simulink model "Hunter_gazebo_sub"  (R2023a)
settings: Solver=ode3  StartTime=0.0  StopTime=inf  FixedStep=0.05  RelTol=1e-3  EnableMultiTasking=on
InitFcn:
  | rosshutdown
  | 
  | rosinit("http://localhost:11311")
  | 
  | load('myfcn.mat');
model workspace (MAT data in the model file):
  SL_ROS_VariableLengthArrays_MaxSizes.CommonInfo.ArrayTruncateAction = 'EmitWarning'
  SL_ROS_VariableLengthArrays_MaxSizes.MsgTypeMap = containers.Map
  SL_ROS_VariableLengthArrays_MaxSizes.MsgTypeMap.serialization.keys = {'cob_object_detection_msgs/Detection', 'cob_object_detection_msgs/DetectionArray', 'cob_perception_msgs/DetectionArray', 'gazebo_msgs/ModelStates', 'sensor_msgs/PointCloud2'}
  SL_ROS_VariableLengthArrays_MaxSizes.MsgTypeMap.serialization.values{1}(1).PropertyName = 'Detector'
  SL_ROS_VariableLengthArrays_MaxSizes.MsgTypeMap.serialization.values{1}(1).DataType = 'uint8'
  SL_ROS_VariableLengthArrays_MaxSizes.MsgTypeMap.serialization.values{1}(1).MaxLength = 128
  SL_ROS_VariableLengthArrays_MaxSizes.MsgTypeMap.serialization.values{1}(2).PropertyName = 'Label'
  SL_ROS_VariableLengthArrays_MaxSizes.MsgTypeMap.serialization.values{1}(2).DataType = 'uint8'
  SL_ROS_VariableLengthArrays_MaxSizes.MsgTypeMap.serialization.values{1}(2).MaxLength = 128
  SL_ROS_VariableLengthArrays_MaxSizes.MsgTypeMap.serialization.values{2}.PropertyName = 'Detections'
  SL_ROS_VariableLengthArrays_MaxSizes.MsgTypeMap.serialization.values{2}.DataType = 'cob_object_detection_msgs/Detection'
  SL_ROS_VariableLengthArrays_MaxSizes.MsgTypeMap.serialization.values{2}.MaxLength = 100
  SL_ROS_VariableLengthArrays_MaxSizes.MsgTypeMap.serialization.values{3}.PropertyName = 'Detections'
  SL_ROS_VariableLengthArrays_MaxSizes.MsgTypeMap.serialization.values{3}.DataType = 'cob_perception_msgs/Detection'
  SL_ROS_VariableLengthArrays_MaxSizes.MsgTypeMap.serialization.values{3}.MaxLength = 50
  SL_ROS_VariableLengthArrays_MaxSizes.MsgTypeMap.serialization.values{4}(1).PropertyName = 'Name'
  SL_ROS_VariableLengthArrays_MaxSizes.MsgTypeMap.serialization.values{4}(1).DataType = 'std_msgs/String'
  SL_ROS_VariableLengthArrays_MaxSizes.MsgTypeMap.serialization.values{4}(1).MaxLength = 266
  SL_ROS_VariableLengthArrays_MaxSizes.MsgTypeMap.serialization.values{4}(2).PropertyName = 'Pose'
  SL_ROS_VariableLengthArrays_MaxSizes.MsgTypeMap.serialization.values{4}(2).DataType = 'geometry_msgs/Pose'
  SL_ROS_VariableLengthArrays_MaxSizes.MsgTypeMap.serialization.values{4}(2).MaxLength = 350
  SL_ROS_VariableLengthArrays_MaxSizes.MsgTypeMap.serialization.values{4}(3).PropertyName = 'Twist'
  SL_ROS_VariableLengthArrays_MaxSizes.MsgTypeMap.serialization.values{4}(3).DataType = 'geometry_msgs/Twist'
  SL_ROS_VariableLengthArrays_MaxSizes.MsgTypeMap.serialization.values{4}(3).MaxLength = 350
  SL_ROS_VariableLengthArrays_MaxSizes.MsgTypeMap.serialization.values{5}(1).PropertyName = 'Data'
  SL_ROS_VariableLengthArrays_MaxSizes.MsgTypeMap.serialization.values{5}(1).DataType = 'uint8'
  SL_ROS_VariableLengthArrays_MaxSizes.MsgTypeMap.serialization.values{5}(1).MaxLength = 1050000
  SL_ROS_VariableLengthArrays_MaxSizes.MsgTypeMap.serialization.values{5}(2).PropertyName = 'Fields'
  SL_ROS_VariableLengthArrays_MaxSizes.MsgTypeMap.serialization.values{5}(2).DataType = 'sensor_msgs/PointField'
  SL_ROS_VariableLengthArrays_MaxSizes.MsgTypeMap.serialization.values{5}(2).MaxLength = 1000
  SL_ROS_VariableLengthArrays_MaxSizes.MsgTypeMap.serialization.uniformity = 0
  SL_ROS_VariableLengthArrays_MaxSizes.MsgTypeMap.serialization.keyType = 'char'
  SL_ROS_VariableLengthArrays_MaxSizes.MsgTypeMap.serialization.valueType = 'any'
values from neighbouring files (symbols this model uses):
  roi = [0, 7, -7, 7, -1, 2]    [TrackExample_sim.m]
undefined symbols (not defined in the file or in its folder): Angular, Linear
libraries: robotlib x7, slpidlib x2, slctrlblks x1, robotalgslib x1, mobileRoboticsLib x1, robotcorelib x1
settings Model: Creator=aiv_  LastModifiedBy=aiv
settings SolverCC: AutoInsertRateTranBlk=on
settings DataIOCC: SaveFormat=Array  ReturnWorkspaceOutputs=off
settings OptimizationCC: EnhancedBackFolding=on  PassReuseOutputArgsAs=Individual arguments  StateBitsets=on  DataBitsets=on  ZeroExternalMemoryAtStartup=off  ZeroInternalMemoryAtStartup=off  NoFixptDivByZeroProtection=on  LifeSpan=1  MaxStackSize=64  OptimizeBlockOrder=speed  DifferentSizesBufferReuse=on  EfficientTunableParamExpr=on
settings DebuggingCC: ParameterTunabilityLossMsg=error
settings HardwareCC: ProdBitPerPointer=32  ProdBitPerSizeT=32  ProdBitPerPtrDiffT=32  ProdLargestAtomicFloat=None  ProdWordSize=32  ProdHWDeviceType=Custom Processor->Custom Processor
settings ModelReferenceCC: PropagateSignalLabelsOutOfModel=off
settings SFSimCC: SimTargetLang=C++
settings RTWCC: Description=Embedded Coder  SystemTargetFile=ert.tlc  HardwareBoard=Robot Operating System (ROS)  TLCOptions=-p0 -aRateBasedStepFcn=0  TemplateMakefile=ert_default_tmf  GenerateReport=on  RTWVerbose=off  Toolchain=Catkin  IncludeHyperlinkInReport=on  LaunchReport=on  TargetLang=C++
settings CodeAppCC: ForceParamTrailComments=on  IgnoreCustomStorageClasses=off  OperatorAnnotations=on  SimulinkDataObjDesc=on  SFDataObjDesc=on  CustomSymbolStrGlobalVar=rt$N$M  CustomSymbolStrType=$N$M  CustomSymbolStrFcn=$N$M$F  CustomSymbolStrMacro=$N$M  InsertBlockDesc=on
settings ERTTargetCC: CodeReplacementLibrary=GNU C99 extensions  SuppressErrorStatus=on  CodeInterfacePackaging=C++ class  SupportVariableSizeSignals=on  RootIOFormat=Structure reference  ERTCustomFileTemplate=example_file_process.tlc

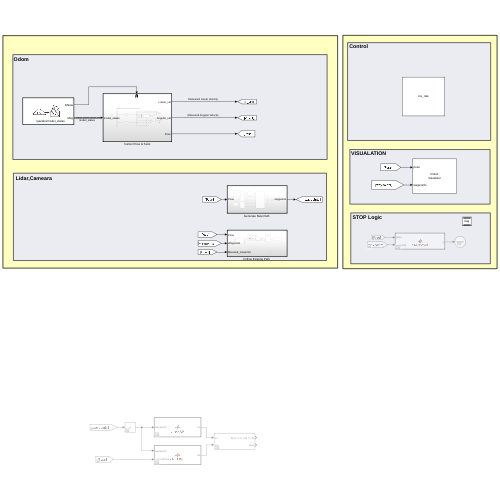
[thumbnail: Simulink's stored preview of the top-level diagram]
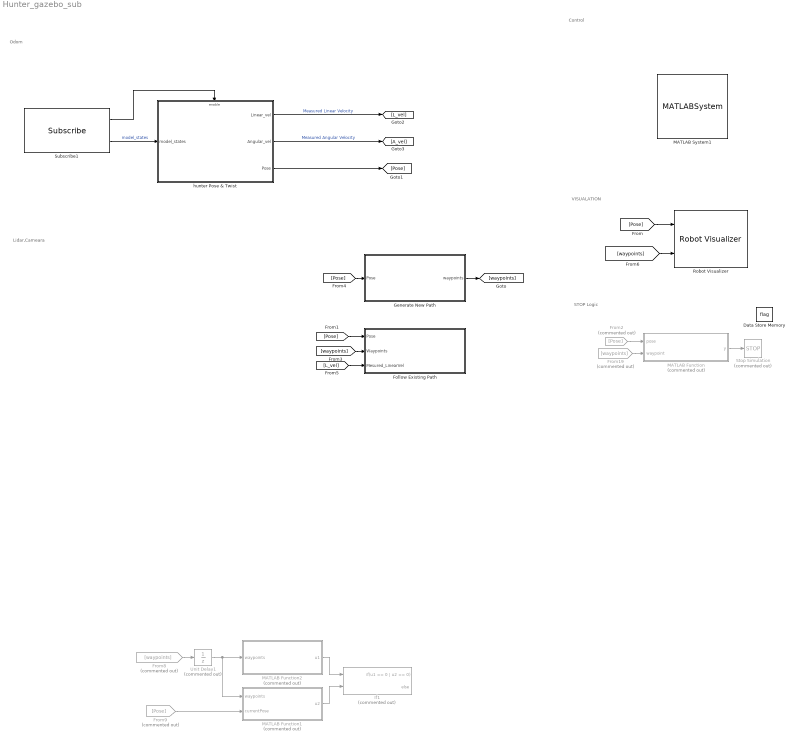
== system Hunter_gazebo_sub ==
  note: VISUALATION
  note: STOP Logic
  note: Odom
  note: Control
  note: Lidar,Cameara
  Data Store Memory : DataStoreMemory  DataStoreName=flag  WriteAfterWriteMsg=warning  ShowAdditionalParam=off  OutDataTypeStr=double
  "Follow Existing Path " : Subsystem  TreatAsAtomicUnit=on
  From19 : From  Commented=on  GotoTag=waypoints
  From2 : From  Commented=on  GotoTag=Pose
  From8 : From  Commented=on  GotoTag=waypoints
  From9 : From  Commented=on  GotoTag=Pose
  "Generate New Path " : Subsystem  TreatAsAtomicUnit=on
  If1 : If  Commented=on  NumInputs=2  IfExpression=u1 == 0 | u2 == 0
  MATLAB Function : MATLAB Function  Commented=on  TreatAsAtomicUnit=on
  MATLAB Function1 : MATLAB Function  Commented=on  TreatAsAtomicUnit=on
  MATLAB Function2 : MATLAB Function  Commented=on  TreatAsAtomicUnit=on
  MATLAB System1 : MATLABSystem  System=ros_rate  RATE=[20]  SimulateUsing=Code generation
      mask Type: ros_rate
      mask Display: disp('ros_rate');
  Robot Visualizer : mobileRoboticsLib/Environments/Robot Visualizer  robotRadius=0  showTrajectory=on  hasWaypoints=on  hasLidar=off  sensorOffset=[ 0, 0 ]  scanAngles=[ -pi/4, 0, pi/4 ]  hasObjDetector=off  objDetectorOffset=[ 0, 0 ]  objDetectorAngle=0  objDetectorFOV=pi/4  objDetectorMaxRange=5  objectColors=[ 1, 0, 0; 0, 1, 0; 0, 0, 1 ]  objectMarkers=s
  Stop Simulation : Stop  Commented=on
  Subscribe1 : robotlib/Subscribe  topicSource=Select from ROS network  topic=/gazebo/model_states  messageType=gazebo_msgs/ModelStates  SampleTime=-1  legacyBusStruct=off  messageQueueLength=1
  Unit Delay1 : UnitDelay  Commented=on  SampleTime=-1  HasFrameUpgradeWarning=on
  hunter Pose & Twist : Subsystem
  wires:
  Subscribe1/1 -> hunter Pose & Twist/Enable
  Subscribe1/2 -> hunter Pose & Twist/1(model_states)  "model_states"
  [waypoints] -> Robot Visualizer/2
  [Pose] -> Robot Visualizer/1
  From2/1 -> MATLAB Function/1(pose)
  MATLAB Function/1(y) -> Stop Simulation/1
  hunter Pose & Twist/1(Linear_vel) -> [L_vel]  "Measured Linear Velocity"
  hunter Pose & Twist/2(Angular_vel) -> [A_vel]  "Measured Angular Velocity"
  From19/1 -> MATLAB Function/2(waypoint)
  [Pose] -> "Generate New Path "/1(Pose)
  "Generate New Path "/1(waypoints) -> [waypoints]
  [Pose] -> "Follow Existing Path "/1(Pose)
  [waypoints] -> "Follow Existing Path "/2(Waypoints)
  [L_vel] -> "Follow Existing Path "/3(Mesured_LinearVel)
  hunter Pose & Twist/3(Pose) -> [Pose]
  MATLAB Function1/1(u2) -> If1/2
  From9/1 -> MATLAB Function1/2(currentPose)
  MATLAB Function2/1(u1) -> If1/1
  Unit Delay1/1 -> MATLAB Function1/1(waypoints), MATLAB Function2/1(waypoints)
  From8/1 -> Unit Delay1/1

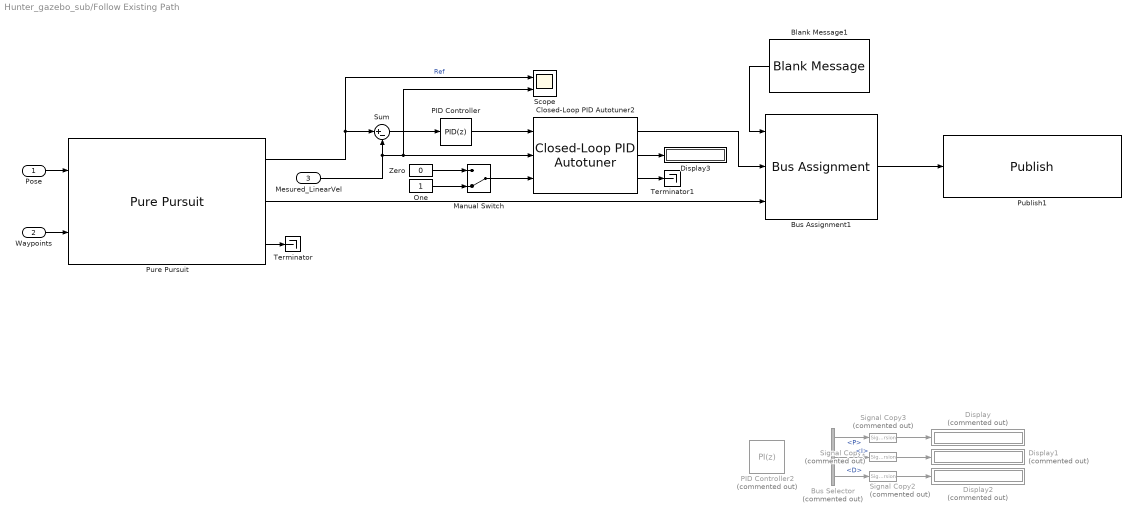
== system Hunter_gazebo_sub/Follow Existing Path  ==
  Pose : Inport
  Waypoints : Inport  Port=2
  Mesured_LinearVel : Inport  Port=3
  Blank Message1 : robotlib/Blank Message  messageClass=Message  entityType=geometry_msgs/Twist  messageType=geometry_msgs/Twist  SampleTime=inf  legacyBusStruct=off
  Bus Assignment1 : BusAssignment  AssignedSignals=Linear.X,Angular.Z
  Bus Selector : BusSelector  Commented=on  OutputSignals=P,I,D
  Closed-Loop PID Autotuner2 : slctrlblks/Closed-Loop PID Autotuner  PIDType=PID  PIDForm=Parallel  TimeDomain=discrete-time  DiscreteTs=0.05  TuningTs=0.2  UseTuningTs=off  IntegratorFormula=Forward Euler  FilterFormula=Forward Euler  ContinuousTs=0.02  Bandwidth=1  UseExternalWC=off  TargetPM=60  UseExternalPM=off  UseExternalAchievedPM=off  ExperimentMode=Superposition  PlantType=Stable  PlantSign=Positive  AmpSine=0.01  UseExternalAmpSine=off  UseExternalFRD=off  UseExternalU0=off  UseCompanion=off  NotDeployTuningModule=off  UsePLCCoder=off  OutputMode=control action + perturbation  BlockDataType=double  UseConnectedPID=on  blockpath=[]  tunedP=0  tunedI=0  tunedD=0  tunedN=100  tunedPM=0  EstimationWindowSize=3  UseExternalTuningParams=off  SingleMultiRateVariant=SingleSamplingRate  NumEstimationPeriods=4  NumSettlingPeriods=2  ExperimentModeVariant=VariantSuperimposed  OutputChoice=VariantCandD
  Display : Display  Commented=on
  Display1 : Display  Commented=on
  Display2 : Display  Commented=on
  Display3 : Display
  Manual Switch : ManualSwitch  CurrentSetting=0
  One : Constant  OutDataTypeStr=Inherit: Inherit via back propagation
  PID Controller : slpidlib/PID Controller  Controller=PID  Form=Parallel  TimeDomain=Discrete-time  UseExternalTs=off  SampleTime=-1  IntegratorMethod=Forward Euler  FilterMethod=Forward Euler  ControllerParametersSource=internal  P=1  I=1  UseKiTs=off  D=0  N=100  UseFilter=on  TunerSelectOption=Transfer Function Based (PID Tuner App)  InitialConditionSource=internal  InitialConditionForIntegrator=0  InitialConditionForFilter=0  DifferentiatorICPrevScaledInput=0  ExternalReset=none  TrackingMode=off  Kt=1  LimitOutput=off  SatLimitsSource=internal  UpperSaturationLimit=inf  LowerSaturationLimit=-inf  LinearizeAsGain=on  AntiWindupMode=none  Kb=1  LimitIntegrator=off  UpperIntegratorSaturationLimit=inf  LowerIntegratorSaturationLimit=-inf  POutMin=[]  POutMax=[]  IOutMin=[]  IOutMax=[]  DOutMin=[]  DOutMax=[]  NOutMin=[]  NOutMax=[]  SumOutMin=[]  SumOutMax=[]  SaturationOutMin=[]  SaturationOutMax=[]  PParamMin=[]  PParamMax=[]  IParamMin=[]  IParamMax=[]  DParamMin=[]  DParamMax=[]  NParamMin=[]  NParamMax=[]  KbParamMin=[]  KbParamMax=[]  KtParamMin=[]  KtParamMax=[]  KbOutMin=[]  KbOutMax=[]  KtOutMin=[]  KtOutMax=[]  IntegratorOutMin=[]  IntegratorOutMax=[]  FilterOutMin=[]  FilterOutMax=[]  SumI1OutMin=[]  SumI1OutMax=[]  SumI2OutMin=[]  SumI2OutMax=[]  SumI3OutMin=[]  SumI3OutMax=[]  SumI4OutMin=[]  SumI4OutMax=[]  SumDOutMin=[]  SumDOutMax=[]  DifferentiatorOutMin=[]  DifferentiatorOutMax=[]  FilterDiffOutCoefMin=[]  FilterDiffOutCoefMax=[]  ReciprocalOutMin=[]  ReciprocalOutMax=[]  SumDenOutMin=[]  SumDenOutMax=[]  SumNumOutMin=[]  SumNumOutMax=[]  DivideOutMin=[]  DivideOutMax=[]  UdiffTsProdOutMin=[]  UdiffTsProdOutMax=[]  NTsProdOutMin=[]  NTsProdOutMax=[]  UintegralTsProdOutMin=[]  UintegralTsProdOutMax=[]  UngainTsProdOutMin=[]  UngainTsProdOutMax=[]  ClampingZeroOutDataTypeStr=Inherit: Inherit via back propagation  ClampingZeroOutMin=[]  ClampingZeroOutMax=[]  FilterDenConstantOutDataTypeStr=Inherit: Inherit via back propagation  FilterDenConstantOutMin=[]  FilterDenConstantOutMax=[]  PCopyOutDataTypeStr=Inherit: Inherit via back propagation  PCopyOutMin=[]  PCopyOutMax=[]  NCopyOutDataTypeStr=Inherit: Inherit via back propagation  NCopyOutMin=[]  NCopyOutMax=[]  IntegratorContinuousStateAttributes=''  IntegratorStateMustResolveToSignalObject=off  IntegratorRTWStateStorageClass=Auto  FilterContinuousStateAttributes=''  FilterStateMustResolveToSignalObject=off  FilterRTWStateStorageClass=Auto  ParallelPVariant=InternalParameters  IdealPVariant=Disabled  IVariant=InternalParameters  DVariant=InternalParameters  IntegratorVariant=Discrete  SatVariant=Disabled  AWVariant=Passthrough  PCopyVariant=Disabled  TRVariant=Disabled  FdbkBlocksVariant=Forward  IdealPFdbkVariant=Disabled  SatFdbkVariant=Disabled  DerivativeFilterVariant=ForwardEulerFilter  NVariant=InternalParameters  NCopyVariant=Disabled  FilterICVariant=InternalICsFilter  IntegratorICVariant=InternalICs  ExternalResetVariant=Disabled  TRSumVariant=Passthrough  SumFdbkVariant=Disabled  SumVariant=Sum_PID  TsampFilterVariant=InternalTs  TsampNgainVariant=Passthrough  TsampIntegralVariant=Disabled_SignalSpec  ExternalSaturationOutDataTypeStr=Inherit: Same as second input
  PID Controller2 : slpidlib/PID Controller  Commented=on  Controller=PI  Form=Parallel  TimeDomain=Discrete-time  UseExternalTs=off  SampleTime=-1  IntegratorMethod=Forward Euler  FilterMethod=Forward Euler  ControllerParametersSource=internal  P=0.6  I=1  UseKiTs=off  D=0.001  N=50  UseFilter=on  TunerSelectOption=Transfer Function Based (PID Tuner App)  InitialConditionSource=internal  InitialConditionForIntegrator=0  InitialConditionForFilter=0  DifferentiatorICPrevScaledInput=0  ExternalReset=none  TrackingMode=off  Kt=1  LimitOutput=off  SatLimitsSource=internal  UpperSaturationLimit=inf  LowerSaturationLimit=-inf  LinearizeAsGain=on  AntiWindupMode=none  Kb=1  LimitIntegrator=off  UpperIntegratorSaturationLimit=inf  LowerIntegratorSaturationLimit=-inf  POutMin=[]  POutMax=[]  IOutMin=[]  IOutMax=[]  DOutMin=[]  DOutMax=[]  NOutMin=[]  NOutMax=[]  SumOutMin=[]  SumOutMax=[]  SaturationOutMin=[]  SaturationOutMax=[]  PParamMin=[]  PParamMax=[]  IParamMin=[]  IParamMax=[]  DParamMin=[]  DParamMax=[]  NParamMin=[]  NParamMax=[]  KbParamMin=[]  KbParamMax=[]  KtParamMin=[]  KtParamMax=[]  KbOutMin=[]  KbOutMax=[]  KtOutMin=[]  KtOutMax=[]  IntegratorOutMin=[]  IntegratorOutMax=[]  FilterOutMin=[]  FilterOutMax=[]  SumI1OutMin=[]  SumI1OutMax=[]  SumI2OutMin=[]  SumI2OutMax=[]  SumI3OutMin=[]  SumI3OutMax=[]  SumI4OutMin=[]  SumI4OutMax=[]  SumDOutMin=[]  SumDOutMax=[]  DifferentiatorOutMin=[]  DifferentiatorOutMax=[]  FilterDiffOutCoefMin=[]  FilterDiffOutCoefMax=[]  ReciprocalOutMin=[]  ReciprocalOutMax=[]  SumDenOutMin=[]  SumDenOutMax=[]  SumNumOutMin=[]  SumNumOutMax=[]  DivideOutMin=[]  DivideOutMax=[]  UdiffTsProdOutMin=[]  UdiffTsProdOutMax=[]  NTsProdOutMin=[]  NTsProdOutMax=[]  UintegralTsProdOutMin=[]  UintegralTsProdOutMax=[]  UngainTsProdOutMin=[]  UngainTsProdOutMax=[]  ClampingZeroOutDataTypeStr=Inherit: Inherit via back propagation  ClampingZeroOutMin=[]  ClampingZeroOutMax=[]  FilterDenConstantOutDataTypeStr=Inherit: Inherit via back propagation  FilterDenConstantOutMin=[]  FilterDenConstantOutMax=[]  PCopyOutDataTypeStr=Inherit: Inherit via back propagation  PCopyOutMin=[]  PCopyOutMax=[]  NCopyOutDataTypeStr=Inherit: Inherit via back propagation  NCopyOutMin=[]  NCopyOutMax=[]  IntegratorContinuousStateAttributes=''  IntegratorStateMustResolveToSignalObject=off  IntegratorRTWStateStorageClass=Auto  FilterContinuousStateAttributes=''  FilterStateMustResolveToSignalObject=off  FilterRTWStateStorageClass=Auto  ParallelPVariant=InternalParameters  IdealPVariant=Disabled  IVariant=InternalParameters  DVariant=Disabled  IntegratorVariant=Discrete  SatVariant=Disabled  AWVariant=Passthrough  PCopyVariant=Disabled  TRVariant=Disabled  FdbkBlocksVariant=Forward  IdealPFdbkVariant=Disabled  SatFdbkVariant=Disabled  DerivativeFilterVariant=Disabled  NVariant=Disabled  NCopyVariant=Disabled_SignalSpec  FilterICVariant=Disabled  IntegratorICVariant=InternalICs  ExternalResetVariant=Disabled  TRSumVariant=Passthrough  SumFdbkVariant=Disabled  SumVariant=Sum_PI  TsampFilterVariant=InternalTs  TsampNgainVariant=Passthrough  TsampIntegralVariant=Disabled_SignalSpec  ExternalSaturationOutDataTypeStr=Inherit: Same as second input
  Publish1 : robotlib/Publish  topicSource=Select from ROS network  topic=/ackermann_steering_controller/cmd_vel  messageType=geometry_msgs/Twist  legacyBusStruct=off  messageQueueLength=1
  Pure Pursuit : robotalgslib/Pure Pursuit  DesiredLinearVelocity=1.5  MaxAngularVelocity=2  LookaheadDistance=1.3  TargetDirPort=on  SimulateUsing=Code generation
      settings: LibrarySourceBlock=navlib/Control Algorithms/Pure Pursuit
  Scope : Scope  NumInputPorts=2
  Signal Copy1 : SignalConversion  Commented=on  OverrideOpt=off
  Signal Copy2 : SignalConversion  Commented=on  OverrideOpt=off
  Signal Copy3 : SignalConversion  Commented=on  OverrideOpt=off
  Sum : Sum  Inputs=|+-
  Terminator : Terminator
  Terminator1 : Terminator
  Zero : Constant  Value=0  OutDataTypeStr=Inherit: Inherit via back propagation
  wires:
  Pose/1 -> Pure Pursuit/1
  Waypoints/1 -> Pure Pursuit/2
  Bus Assignment1/1 -> Publish1/1
  Blank Message1/1 -> Bus Assignment1/1
  Pure Pursuit/3 -> Terminator/1
  Pure Pursuit/2 -> Bus Assignment1/3
  Pure Pursuit/1 -> Scope/1, Sum/1  "Ref"
  Sum/1 -> PID Controller/1
  Closed-Loop PID Autotuner2/2 -> Display3/1
  One/1 -> Manual Switch/2
  Zero/1 -> Manual Switch/1
  Manual Switch/1 -> Closed-Loop PID Autotuner2/3
  Mesured_LinearVel/1 -> Scope/2, Closed-Loop PID Autotuner2/2, Sum/2
  PID Controller/1 -> Closed-Loop PID Autotuner2/1
  Bus Selector/3 -> Signal Copy2/1  "<D>"
  Bus Selector/2 -> Signal Copy1/1  "<I>"
  Signal Copy2/1 -> Display2/1
  Signal Copy1/1 -> Display1/1
  Bus Selector/1 -> Signal Copy3/1  "<P>"
  Signal Copy3/1 -> Display/1
  Closed-Loop PID Autotuner2/3 -> Terminator1/1
  Closed-Loop PID Autotuner2/1 -> Bus Assignment1/2

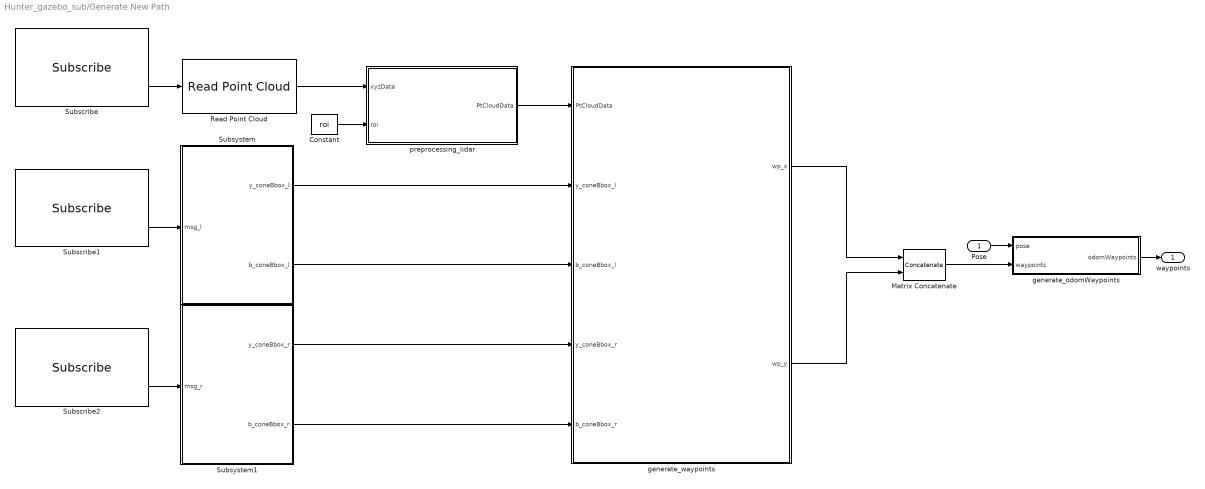
== system Hunter_gazebo_sub/Generate New Path  ==
  Pose : Inport
  Constant : Constant  Value=roi
  Matrix Concatenate : Concatenate  Mode=Multidimensional array  ConcatenateDimension=2
  Read Point Cloud : robotlib/Read Point Cloud  MaximumPointCloudSize=[1, 32768]  PreserveStructure=on  ShowRGBOutput=off  ShowIntensityOutput=off  ShowErrorCodeOutput=off  VariableSizeOutputs=off
  Subscribe : robotlib/Subscribe  topicSource=Select from ROS network  topic=/lidar  messageType=sensor_msgs/PointCloud2  SampleTime=-1  legacyBusStruct=off  messageQueueLength=1
  Subscribe1 : robotlib/Subscribe  topicSource=Select from ROS network  topic=/yolov5/cob_detections_l  messageType=cob_perception_msgs/DetectionArray  SampleTime=-1  legacyBusStruct=off  messageQueueLength=1
  Subscribe2 : robotlib/Subscribe  topicSource=Select from ROS network  topic=/yolov5/cob_detections_r  messageType=cob_perception_msgs/DetectionArray  SampleTime=-1  legacyBusStruct=off  messageQueueLength=1
  Subsystem : Subsystem
  Subsystem1 : Subsystem
  generate_odomWaypoints : MATLAB Function  TreatAsAtomicUnit=on
  generate_waypoints : MATLAB Function  TreatAsAtomicUnit=on
  preprocessing_lidar : MATLAB Function  TreatAsAtomicUnit=on
  waypoints : Outport
  wires:
  generate_odomWaypoints/1(odomWaypoints) -> waypoints/1
  Pose/1 -> generate_odomWaypoints/1(pose)
  Constant/1 -> preprocessing_lidar/2(roi)
  preprocessing_lidar/1(PtCloudData) -> generate_waypoints/1(PtCloudData)
  Subscribe/2 -> Read Point Cloud/1
  Subscribe1/2 -> Subsystem/1(msg_l)
  Subscribe2/2 -> Subsystem1/1(msg_r)
  Read Point Cloud/1 -> preprocessing_lidar/1(xyzData)
  Subsystem/1(y_coneBbox_l) -> generate_waypoints/2(y_coneBbox_l)
  Subsystem/2(b_coneBbox_l) -> generate_waypoints/3(b_coneBbox_l)
  Subsystem1/1(y_coneBbox_r) -> generate_waypoints/4(y_coneBbox_r)
  Subsystem1/2(b_coneBbox_r) -> generate_waypoints/5(b_coneBbox_r)
  Matrix Concatenate/1 -> generate_odomWaypoints/2(waypoints)
  generate_waypoints/1(wp_x) -> Matrix Concatenate/1
  generate_waypoints/2(wp_y) -> Matrix Concatenate/2

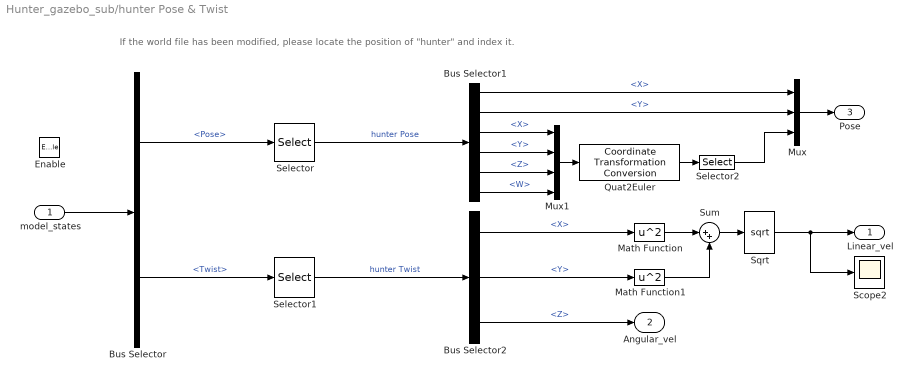
== system Hunter_gazebo_sub/hunter Pose & Twist ==
  note: If the world file has been modified, please locate the position of "hunter" and index it.
  model_states : Inport
  Enable : EnablePort  StatesWhenEnabling=reset
  Bus Selector : BusSelector  OutputSignals=Pose,Twist
  Bus Selector1 : BusSelector  OutputSignals=Position.X,Position.Y,Orientation.X,Orientation.Y,Orientation.Z,Orientation.W
  Bus Selector2 : BusSelector  OutputSignals=Linear.X,Linear.Y,Angular.Z
  Math Function : Math  Operator=square
  Math Function1 : Math  Operator=square
  Mux : Mux  Inputs=3
  Mux1 : Mux
  Quat2Euler : robotcorelib/Coordinate Transformation Conversion  InputRepresentation=Quaternion  InputEulerSequence=ZYX  ShowTrVecInputPort=on  OutputRepresentation=Euler Angles  OutputEulerSequence=ZYX  ShowTrVecOutputPort=on  SimulateUsing=Interpreted execution
  Scope2 : Scope
  Selector : Selector  InputPortWidth=350  IndexOptions=Index vector (dialog)  Indices=137  OutputSizes=1
  Selector1 : Selector  InputPortWidth=350  IndexOptions=Index vector (dialog)  Indices=[137]  OutputSizes=1
  Selector2 : Selector  InputPortWidth=3  IndexOptions=Index vector (dialog)  Indices=3  OutputSizes=1
  Sqrt : Sqrt
  Sum : Sum  Inputs=|++
  Linear_vel : Outport
  Angular_vel : Outport  Port=2
  Pose : Outport  Port=3
  wires:
  model_states/1 -> Bus Selector/1
  Bus Selector1/5 -> Mux1/3  "<Z>"
  Bus Selector1/3 -> Mux1/1  "<X>"
  Selector/1 -> Bus Selector1/1  "hunter Pose"
  Bus Selector1/6 -> Mux1/4  "<W>"
  Bus Selector2/1 -> Math Function/1  "<X>"
  Bus Selector1/4 -> Mux1/2  "<Y>"
  Selector1/1 -> Bus Selector2/1  "hunter Twist"
  Bus Selector1/1 -> Mux/1  "<X>"
  Bus Selector1/2 -> Mux/2  "<Y>"
  Bus Selector/1 -> Selector/1  "<Pose>"
  Bus Selector/2 -> Selector1/1  "<Twist>"
  Selector2/1 -> Mux/3
  Sum/1 -> Sqrt/1
  Bus Selector2/2 -> Math Function1/1  "<Y>"
  Math Function/1 -> Sum/1
  Math Function1/1 -> Sum/2
  Sqrt/1 -> Linear_vel/1, Scope2/1
  Bus Selector2/3 -> Angular_vel/1  "<Z>"
  Mux/1 -> Pose/1
  Mux1/1 -> Quat2Euler/1
  Quat2Euler/1 -> Selector2/1

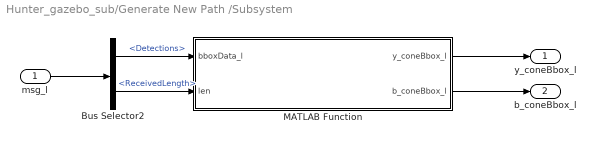
== system Hunter_gazebo_sub/Generate New Path /Subsystem ==
  msg_l : Inport
  Bus Selector2 : BusSelector  OutputSignals=Detections,Detections_SL_Info.ReceivedLength
  MATLAB Function : MATLAB Function  TreatAsAtomicUnit=on
  y_coneBbox_l : Outport
  b_coneBbox_l : Outport  Port=2
  wires:
  msg_l/1 -> Bus Selector2/1
  Bus Selector2/1 -> MATLAB Function/1(bboxData_l)  "<Detections>"
  MATLAB Function/1(y_coneBbox_l) -> y_coneBbox_l/1
  MATLAB Function/2(b_coneBbox_l) -> b_coneBbox_l/1
  Bus Selector2/2 -> MATLAB Function/2(len)  "<ReceivedLength>"

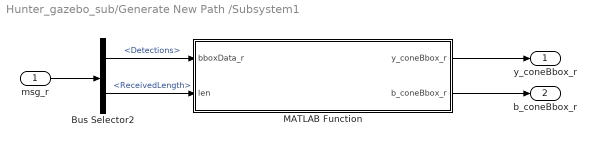
== system Hunter_gazebo_sub/Generate New Path /Subsystem1 ==
  msg_r : Inport
  Bus Selector2 : BusSelector  OutputSignals=Detections,Detections_SL_Info.ReceivedLength
  MATLAB Function : MATLAB Function  TreatAsAtomicUnit=on
  y_coneBbox_r : Outport
  b_coneBbox_r : Outport  Port=2
  wires:
  msg_r/1 -> Bus Selector2/1
  Bus Selector2/1 -> MATLAB Function/1(bboxData_r)  "<Detections>"
  MATLAB Function/1(y_coneBbox_r) -> y_coneBbox_r/1
  MATLAB Function/2(b_coneBbox_r) -> b_coneBbox_r/1
  Bus Selector2/2 -> MATLAB Function/2(len)  "<ReceivedLength>"

== matlab function Hunter_gazebo_sub/MATLAB Function1 ==
  data: waypoints input; u2 output; currentPose input
function u2 = checkDist(waypoints, currentPose)

   if norm(waypoints(end,:) - [currentPose(1) currentPose(2)]) < 2
       u2 = 0;  % generate new waypoints
   else
       u2 = 1;  % follow existing waypoints
   end

== matlab function Hunter_gazebo_sub/MATLAB Function ==
  data: pose input; y output; waypoint input; flag data_store_memory
function y = CheckPoint(pose,waypoint)
    
    hunter_x = pose(1);
    hunter_y = pose(2);
    goalPoint = waypoint(end,:);
    global flag
    
    
    checkWp = waypoint(117:155,:);
    checkWp_x = checkWp(:,1);
    checkWp_y = checkWp(:,2);
    
    max_x = max(checkWp_x);
    min_x = min(checkWp_x);
    max_y = max(checkWp_y);
    min_y = min(checkWp_y);

    if (min_x <= hunter_x && hunter_x <= max_x) && (min_y <= hunter_y && hunter_y <= max_y) 
        flag = 1;
    end
    
    distance = sqrt((hunter_x - goalPoint(1))^2 + (hunter_y - goalPoint(2))^2);

    if (flag ~= 0) && (distance <= 0.65) 
        y = 1;
        disp("Stop Simulation !");
    else
        y = 0;
    end

end

== matlab function Hunter_gazebo_sub/MATLAB Function2 ==
  data: waypoints input; u1 output
function u1 = checkWP(waypoints)
    
        
    if isempty(find(waypoints))
        u1 = 0;  % generate new waypoint
    else
        u1 = 1;  % follow existing waypoint
    end

end

== matlab function Hunter_gazebo_sub/Generate New Path /preprocessing_lidar ==
  data: xyzData input single; roi input; PtCloudData output size=[3000 3]
function PtCloudData = preprocessing_lidar(xyzData,roi)
    % waypoint_x, waypoint_y
    %% preprocessing raw lidar data
    params = lidarParameters('OS1Gen1-64',512);

    ptCloud = pointCloud(xyzData);
    ptCloudOrg = pcorganize(ptCloud,params);
    
    groundPtIdx = segmentGroundFromLidarData(ptCloudOrg);
    nonGroundPtCloud = select(ptCloudOrg,~groundPtIdx,'OutputSize','full');
    
    indices = findPointsInROI(nonGroundPtCloud,roi);
    roiPtCloud = select(nonGroundPtCloud,indices);

    roiPtCloud = pcdenoise(roiPtCloud,"PreserveStructure",true);
    PtCloudData = roiPtCloud.Location;
    
end

== matlab function Hunter_gazebo_sub/Generate New Path /Subsystem/MATLAB Function ==
  data: bboxData_l input; y_coneBbox_l output size=[60,4]; b_coneBbox_l output size=[60,4]; len input
function [y_coneBbox_l, b_coneBbox_l] = extractConesBboxs(bboxData_l,len)

    temp_y_coneBboxs = zeros(len, 4);
    temp_b_coneBboxs = zeros(len, 4);
    y_count = 0;
    b_count = 0;

    for i = 1:len
        x = bboxData_l(i).Mask.Roi.X;
        y = bboxData_l(i).Mask.Roi.Y;
        w = bboxData_l(i).Mask.Roi.Width;
        h = bboxData_l(i).Mask.Roi.Height;
        st = char((bboxData_l(i).Label)');
        if strcmp(st(:,1:6),'y_cone')
            y_count = y_count + 1;
            temp_y_coneBboxs(y_count,:) = [x y w h];
        elseif strcmp(st(:,1:6),'b_cone')
            b_count = b_count + 1;
            temp_b_coneBboxs(b_count,:) = [x y w h];
        else
            disp("extract cone err\n");
        end
    end

    y_coneBbox_l = temp_y_coneBboxs(1:y_count, :);
    b_coneBbox_l = temp_b_coneBboxs(1:b_count, :);

end

== matlab function Hunter_gazebo_sub/Generate New Path /generate_waypoints ==
  data: PtCloudData input single size=[3000 3]; y_coneBbox_l input; b_coneBbox_l input; y_coneBbox_r input; b_coneBbox_r input; wp_x output size=[50,1]; wp_y output size=[50,1]
function [wp_x, wp_y] = generate_waypoints(PtCloudData, y_coneBbox_l, b_coneBbox_l,y_coneBbox_r, b_coneBbox_r)
    

    % tic
    %#codegen
    coder.extrinsic("FinalFulltrack");
    wp_x = double(zeros(50,1));
    wp_y = double(zeros(50,1));


    [wp_x, wp_y] = FinalFulltrack(PtCloudData, y_coneBbox_l, b_coneBbox_l, y_coneBbox_r, b_coneBbox_r);
    % disp(toc)
   
end

== matlab function Hunter_gazebo_sub/Generate New Path /generate_odomWaypoints ==
  data: pose input; waypoints input; odomWaypoints output double size=[50,2]
function odomWaypoints = fcn(pose, waypoints)
    % Initialize transformed waypoints
    odomWaypoints = zeros(size(waypoints));
    % odomWaypoints = zeros(3,2);
    
    % Extract the vehicle's yaw angle
    theta = pose(3);

    % Create the 2D rotation matrix
    R = [cos(theta), -sin(theta);
         sin(theta), cos(theta)];

    % Transform each waypoint
    for i = 1:size(waypoints,1)
        % Rotate the waypoint considering the vehicle's yaw
        rotatedPoint = R * waypoints(i,:)';

        % Translate considering the vehicle's position in the odom frame
        odomWaypoints(i,:) = rotatedPoint' + pose(1:2)';
    end
    
    
end

== matlab function Hunter_gazebo_sub/Generate New Path /Subsystem1/MATLAB Function ==
  data: bboxData_r input; y_coneBbox_r output size=[60,4]; b_coneBbox_r output size=[60,4]; len input
function [y_coneBbox_r, b_coneBbox_r] = extractConesBboxs(bboxData_r,len)
   
    temp_y_coneBboxs = zeros(len, 4);
    temp_b_coneBboxs = zeros(len, 4);
    y_count = 0;
    b_count = 0;

    for i = 1:len
        x = bboxData_r(i).Mask.Roi.X;
        y = bboxData_r(i).Mask.Roi.Y;
        w = bboxData_r(i).Mask.Roi.Width;
        h = bboxData_r(i).Mask.Roi.Height;
        st = char((bboxData_r(i).Label)');
        if strcmp(st(:,1:6), 'y_cone')
            y_count = y_count + 1;
            temp_y_coneBboxs(y_count,:) = [x y w h];
        elseif strcmp(st(:,1:6), 'b_cone')
            b_count = b_count + 1;
            temp_b_coneBboxs(b_count,:) = [x y w h];
        else
            disp("extract cone err\n");
        end
    end

    y_coneBbox_r = temp_y_coneBboxs(1:y_count, :);
    b_coneBbox_r = temp_b_coneBboxs(1:b_count, :);
end
